simulink model "sedemo_rateestimator_initialdesign"  (Simulink 7.5)
settings: Solver=VariableStepDiscrete  StartTime=0.0  StopTime=1200  MaxStep=inf  RelTol=1e-3
libraries: simeventssink1 x4, simeventstranslate1 x1, simeventsgenerators1 x1, simeventsinfo x1, simeventsrouting1 x1, simulink x1
settings Model: Creator=The MathWorks Inc.
settings DataIOCC: SaveOutput=off  SaveTime=off
settings OptimizationCC: InitFltsAndDblsToZero=on  EfficientMapNaN2IntZero=off
settings DebuggingCC: AlgebraicLoopMsg=error  SolverPrmCheckMsg=none  StrictBusMsg=Warning
settings SimEventsCC: propDiagAttribOutput=1  propDiagFcnCallOutput=1  propDiagStatOutput=0

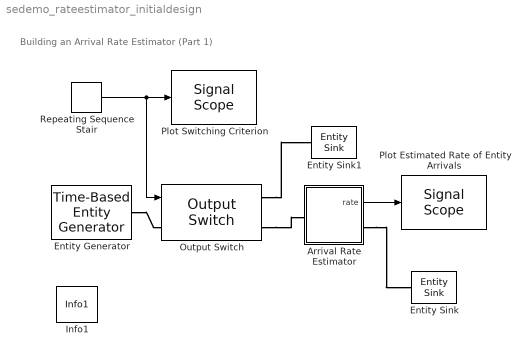
== system sedemo_rateestimator_initialdesign ==
  note: Building an Arrival Rate Estimator (Part 1)
  Arrival Rate Estimator : Subsystem  mask(Rate Estimator){p=0.1}
      mask prompts: p "Smoothing factor p (0<p<1):"
      mask help: Estimate number of arriving entities per second, where p is a smoothing factor that determines how much weight is given to the old estimate. If p is near 0, the estimate is more sensitive. If p is near 1, the estimate is smoother.
  Entity Generator : simeventsgenerators1/Entity Generators/Time-Based Entity Generator  Priority=1  DialogController=des_ddg_create  DialogControllerArgs=DataTag2  SystemSampleTime=-1  GenerateEntitiesUpon=Intergeneration time from dialog  Distribution=Constant  Minimum=0  Maximum=1  Mean=1  InitialSeed=12345  Period=4  PriorityEntityGeneration=300  GenerateEntityAtSimulationStart=off  ResponseWhenBlocked=Pause generation  ResponseWhenUnblocked=Immediate restart  EntityType=Standard  StatNumberDeparted=Off  StatPendingEntity=Off  StatAverageIntergenerationTime=Off
      settings: AttributesFormatString=Period = %<Period>
  Entity Sink : simeventssink1/Entity Sink  Priority=1  SystemSampleTime=-1  AvailableForArrivals=on  StatNumberArrived=Off
  Entity Sink1 : simeventssink1/Entity Sink  Priority=1  SystemSampleTime=-1  AvailableForArrivals=on  StatNumberArrived=Off
  Info1 : simeventsinfo/Info1  SystemSampleTime=-1  file_name=sedemo_rateestimator_m
  Output Switch : simeventsrouting1/Output Switch  Priority=1  SystemSampleTime=-1  NumberOutputPorts=2  SwitchingCriterion=From signal port p  InitialSeed=34567  AttributeName=Attribute1  InitialConditionsOpt=on  InitialConditions=1  EntityBufferOpt=off  SpecifyEventPriority=off  PriorityOutputSwitchSelectPort=4100  TimeoutPortOpt=off  StatNumberDeparted=Off  StatNumberTimedOut=Off  StatPendingEntity=Off  StatLastDeparturePort=Off  EvaluatedNumPorts=2
  Plot Estimated Rate of Entity Arrivals : simeventssink1/Signal Scope  Priority=1  SystemSampleTime=-1  PlotType=Continuous  InputType=Signal  NumInputs=1  AttributeNameY=Count  XInputOptionSignal=Event time  XInputOptionEntity=Event time  AttributeNameX=Count  EnableEntityOutport=on  XMin=-3  XMax=1203  XLimitExceededOption=Stretch axis limits  YLimitExceededOption=Stretch axis limits  AxisGrid=on  AxisLegend=off  LineDisables=""  LineColors="0  0  1"  LineStyles=-  LineMarkers=.  OpenScopeAtSimStart=on  Title=Arrival Rate Estimated Upon Arrivals  YLabel=""  XLabel=Time  FigurePosition=[543 201 438 210]  AxisZoom=off  DataStoreOption=Limited  DataPointsLimit=10000  StatNumberArrived=Off  ShowCountPlotted=off  ShowToolbar=on
      settings: YMin=-0.005  YMax=.3
  Plot Switching Criterion : simeventssink1/Signal Scope  Priority=1  SystemSampleTime=-1  PlotType=Stair  InputType=Signal  NumInputs=1  AttributeNameY=Count  XInputOptionSignal=Event time  XInputOptionEntity=Event time  AttributeNameX=Count  EnableEntityOutport=on  XMin=-3  XMax=1203  XLimitExceededOption=Stretch axis limits  YLimitExceededOption=Keep axis limits unchanged  AxisGrid=off  AxisLegend=off  LineDisables=""  LineColors="1  0  0"  LineStyles=-  LineMarkers=.  OpenScopeAtSimStart=on  Title=Switching Criterion (p=2 is through rate estimator)  YLabel=""  XLabel=Time  FigurePosition=[543 487 438 210]  AxisZoom=off  DataStoreOption=Limited  DataPointsLimit=10000  StatNumberArrived=Off  ShowCountPlotted=off  ShowToolbar=on
      settings: YMin=0.9  YMax=2.1
  Repeating Sequence Stair : simulink/Sources/Repeating Sequence Stair  SystemSampleTime=-1  OutValues=[2 1 2 1]  tsamp=200  OutMin=[]  OutMax=[]  OutDataTypeStr=float('double')  OutputDataTypeScalingMode=Specify via dialog  OutDataType=float('double')  ConRadixGroup=Best Precision: Vector-wise  OutScaling=2^-12
  wires:
  Arrival Rate Estimator/1(rate) -> Plot Estimated Rate of Entity Arrivals/1
  Repeating Sequence Stair/1 -> Output Switch/1, Plot Switching Criterion/1
  connections:
  Entity Generator/RConn1 -- Output Switch/LConn1
  Output Switch/RConn1 -- Entity Sink1/LConn1
  Output Switch/RConn2 -- Arrival Rate Estimator/LConn1
  Arrival Rate Estimator/RConn1 -- Entity Sink/LConn1

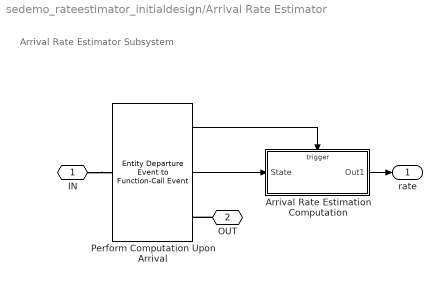
== system sedemo_rateestimator_initialdesign/Arrival Rate Estimator ==
  note: Arrival Rate Estimator Subsystem
  Arrival Rate Estimation Computation : Subsystem  TreatAsAtomicUnit=on
      settings: PropExecContextOutsideSubsystem=on
  Perform Computation Upon Arrival : simeventstranslate1/Entity Departure Event to Function-Call Event  Priority=1  SystemSampleTime=-1  TimingFunctionCallF1=After entity departure  EnableE1Port=off  EnableF2Port=off  TimingFunctionCallF2=After entity departure  EnableE2Port=off  StatNumberDeparted=Off  StatNumberF1Calls=On  StatNumberF2Calls=Off  IsInsideAFB=off
  IN : PMIOPort  Port=1  Side=Left
  OUT : PMIOPort  Port=2  Side=Right
  rate : Outport  OutDataType=sfix(16)  OutScaling=2^0
  wires:
  Arrival Rate Estimation Computation/1(Out1) -> rate/1
  Perform Computation Upon Arrival/2 -> Arrival Rate Estimation Computation/1(State)
  Perform Computation Upon Arrival/1 -> Arrival Rate Estimation Computation/Trigger
  connections:
  IN/RConn1 -- Perform Computation Upon Arrival/LConn1
  OUT/RConn1 -- Perform Computation Upon Arrival/RConn1

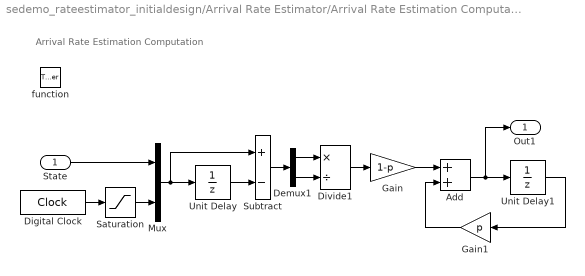
== system sedemo_rateestimator_initialdesign/Arrival Rate Estimator/Arrival Rate Estimation Computation ==
  note: Arrival Rate Estimation Computation
  State : Inport  OutDataType=sfix(16)  OutScaling=2^0
  function : TriggerPort  TriggerType=function-call
  Add : Sum  OutDataType=sfix(16)  OutScaling=2^-10
  Demux1 : Demux  Outputs=2
  Digital Clock : DigitalClock  SampleTime=-1
  Divide1 : Product  Inputs=*/  OutDataType=sfix(16)  OutScaling=2^-10
  Gain : Gain  Gain=1-p  ParameterDataType=sfix(16)  ParameterScaling=2^0  OutDataType=sfix(16)  OutScaling=2^0
  Gain1 : Gain  Gain=p  ParameterDataType=sfix(16)  ParameterScaling=2^0  OutDataType=sfix(16)  OutScaling=2^0
  Mux : Mux  Inputs=2
  Saturation : Saturate  UpperLimit=inf  LowerLimit=1e-5  ZeroCross=off  OutDataType=sfix(16)  OutScaling=2^0
  Subtract : Sum  Inputs=+-  OutDataType=sfix(16)  OutScaling=2^-10
  Unit Delay : UnitDelay  SampleTime=-1
  Unit Delay1 : UnitDelay  SampleTime=-1
  Out1 : Outport  OutDataType=sfix(16)  OutScaling=2^0
  wires:
  Mux/1 -> Subtract/1, Unit Delay/1
  Gain/1 -> Add/1
  State/1 -> Mux/1
  Unit Delay/1 -> Subtract/2
  Unit Delay1/1 -> Gain1/1
  Gain1/1 -> Add/2
  Add/1 -> Unit Delay1/1, Out1/1
  Subtract/1 -> Demux1/1
  Demux1/1 -> Divide1/1
  Demux1/2 -> Divide1/2
  Divide1/1 -> Gain/1
  Digital Clock/1 -> Saturation/1
  Saturation/1 -> Mux/2
